simulink model "washout"  (R2014b)
settings: Solver=ode3  StartTime=0.0  StopTime=Time(end)  FixedStep=0.01  RelTol=1e-3
values from neighbouring files (symbols this model uses):
  K_smooth = 0.1    [UKF_start.m]
  K_smooth_2 = 10    [UKF_start.m]
  K_yaw_diff = 0    [UKF_start.m]
  rollGrad = 5*(pi/180)    (= 0.0872664625997)    [Init_for_washout_filter.m]    (also in Init_for_washout_filter2.m; Init_for_washout_filter3.m; Init_for_washout_filter4.m; UKF_start.m)
  squared = 1    [UKF_start.m]
  T = 0.4    [UKF_start.m]
settings Model: Creator=eric  LastModifiedBy=eric

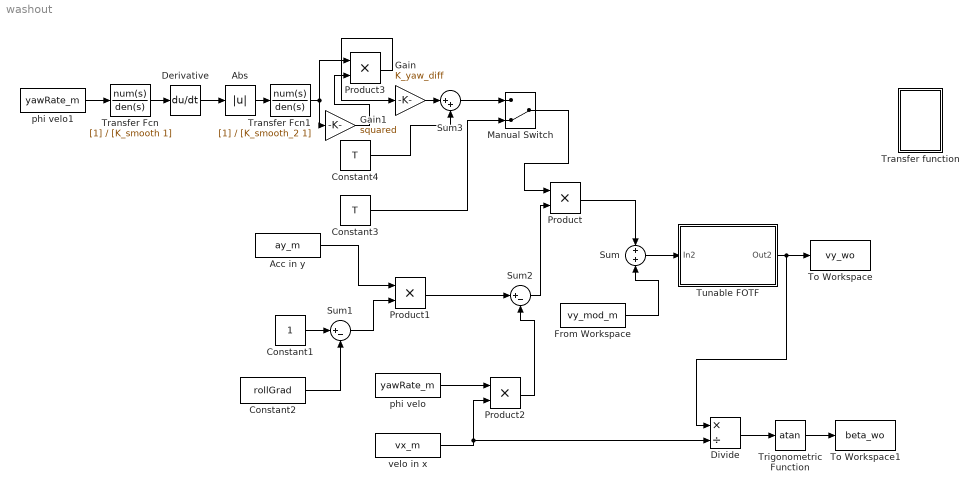
== system washout ==
  Abs : Abs
  Acc in y : FromWorkspace  VariableName=ay_m  SampleTime=0.01
  Constant1 : Constant
  Constant2 : Constant  Value=rollGrad
  Constant3 : Constant  Value=T
  Constant4 : Constant  Value=T
  Derivative : Derivative
  Divide : Product  Inputs=*/
  From Workspace : FromWorkspace  VariableName=vy_mod_m  SampleTime=0.01
  Gain : Gain  Gain=K_yaw_diff
  Gain1 : Gain  Gain=squared
  Manual Switch : ManualSwitch  CurrentSetting=0
  Product{,1..3} (4 alike) : Product
  Sum : Sum
  Sum1 : Sum  Inputs=|+-
  Sum2 : Sum  Inputs=|+-
  Sum3 : Sum  Inputs=|++
  To Workspace : ToWorkspace  VariableName=vy_wo  SaveFormat=Timeseries  SampleTime=-1
  To Workspace1 : ToWorkspace  VariableName=beta_wo  SaveFormat=Timeseries  SampleTime=-1
  Transfer Fcn : TransferFcn  Denominator=[K_smooth 1]
  Transfer Fcn1 : TransferFcn  Denominator=[K_smooth_2 1]
  Transfer function : Subsystem
  Trigonometric Function : Trigonometry  Operator=atan
  Tunable FOTF : Subsystem  mask{a=T}
      mask Display: disp(strvcat(['  1'],['------'],['s + a']))
  phi velo : FromWorkspace  VariableName=yawRate_m  SampleTime=0.01
  phi velo1 : FromWorkspace  VariableName=yawRate_m  SampleTime=0.01
  velo in x : FromWorkspace  VariableName=vx_m  SampleTime=0.01
  wires:
  Manual Switch/1 -> Product/1
  Constant1/1 -> Sum1/1
  Constant2/1 -> Sum1/2
  Sum1/1 -> Product1/2
  Acc in y/1 -> Product1/1
  Product1/1 -> Sum2/1
  Sum2/1 -> Product/2
  phi velo/1 -> Product2/1
  velo in x/1 -> Divide/2, Product2/2
  Product2/1 -> Sum2/2
  Product/1 -> Sum/1
  From Workspace/1 -> Sum/2
  Divide/1 -> Trigonometric Function/1
  Trigonometric Function/1 -> To Workspace1/1
  Sum/1 -> Tunable FOTF/1(In2)
  Tunable FOTF/1(Out2) -> Divide/1, To Workspace/1
  phi velo1/1 -> Transfer Fcn/1
  Constant4/1 -> Sum3/2
  Sum3/1 -> Manual Switch/1
  Constant3/1 -> Manual Switch/2
  Gain/1 -> Sum3/1
  Transfer Fcn/1 -> Derivative/1
  Derivative/1 -> Abs/1
  Abs/1 -> Transfer Fcn1/1
  Transfer Fcn1/1 -> Product3/1, Gain1/1
  Gain1/1 -> Product3/2
  Product3/1 -> Gain/1

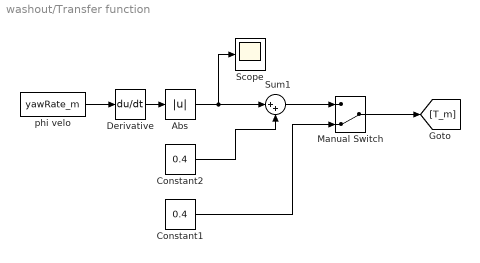
== system washout/Transfer function ==
  Abs : Abs
  Constant1 : Constant  Value=0.4
  Constant2 : Constant  Value=0.4
  Derivative : Derivative
  Manual Switch : ManualSwitch  CurrentSetting=0
  Scope : Scope
  Sum1 : Sum  Inputs=|++
  phi velo : FromWorkspace  VariableName=yawRate_m  SampleTime=0.01
  wires:
  Manual Switch/1 -> [T_m]
  phi velo/1 -> Derivative/1
  Derivative/1 -> Abs/1
  Constant2/1 -> Sum1/2
  Sum1/1 -> Manual Switch/1
  Constant1/1 -> Manual Switch/2
  Abs/1 -> Scope/1, Sum1/1

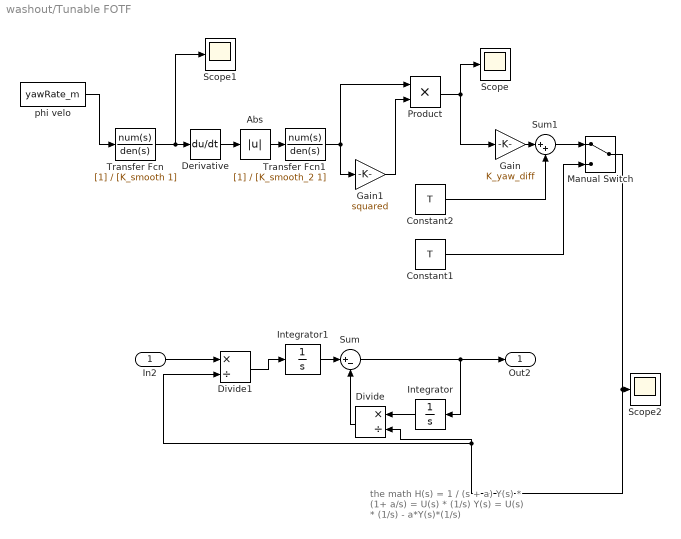
== system washout/Tunable FOTF ==
  note: the math
      | H(s) = 1 /  (s + a)
      | Y(s) * (1+ a/s) = U(s) * (1/s)
      | Y(s) = U(s) * (1/s) - a*Y(s)*(1/s)
  In2 : Inport
  Abs : Abs
  Constant1 : Constant  Value=T
  Constant2 : Constant  Value=T
  Derivative : Derivative
  Divide : Product  Inputs=*/
  Divide1 : Product  Inputs=*/
  Gain : Gain  Gain=K_yaw_diff
  Gain1 : Gain  Gain=squared
  Integrator : Integrator
  Integrator1 : Integrator
  Manual Switch : ManualSwitch
  Product : Product
  Scope : Scope
      settings: SaveName=ScopeData2
  Scope1 : Scope
      settings: TimeRange=30.04
  Scope2 : Scope
      settings: SaveName=ScopeData3
  Sum : Sum  Inputs=|+-
  Sum1 : Sum  Inputs=|++
  Transfer Fcn : TransferFcn  Denominator=[K_smooth 1]
  Transfer Fcn1 : TransferFcn  Denominator=[K_smooth_2 1]
  phi velo : FromWorkspace  VariableName=yawRate_m  SampleTime=0.01
  Out2 : Outport
  wires:
  Integrator/1 -> Divide/1
  Divide/1 -> Sum/2
  Sum/1 -> Integrator/1, Out2/1
  Integrator1/1 -> Sum/1
  Manual Switch/1 -> Scope2/1, Divide/2, Divide1/2
  In2/1 -> Divide1/1
  Divide1/1 -> Integrator1/1
  phi velo/1 -> Transfer Fcn/1
  Constant2/1 -> Sum1/2
  Sum1/1 -> Manual Switch/1
  Constant1/1 -> Manual Switch/2
  Gain/1 -> Sum1/1
  Transfer Fcn/1 -> Scope1/1, Derivative/1
  Derivative/1 -> Abs/1
  Abs/1 -> Transfer Fcn1/1
  Transfer Fcn1/1 -> Product/1, Gain1/1
  Gain1/1 -> Product/2
  Product/1 -> Gain/1, Scope/1
